simulink model "SF105A_MotCurrRegVltgLimr"  (R2013b)
settings: Solver=FixedStepDiscrete  SolverMode=SingleTasking  StartTime=0.0  StopTime=1  FixedStep=0.00025  RelTol=1e-3
undefined symbols (not defined in the file): ARCHGLBPRM_2OVERSQRT3_ULS_F32, ARCHGLBPRM_2PI_ULS_F32, BRDGVLTGHILIM_VOLT_F32, ELECGLBPRM_PWMPERDNOMX2_SEC_F32, F32TOU16OVR2PI_ULS_F32, MotCurrRegCfgCurrLoopSecOrderTrfFctEna, MotCurrRegCfgMotRVirtDax, MotCurrRegCfgMotRVirtQax, MotCurrRegVltgLimrCurrLoaScarSlewRate, MotCurrRegVltgLimrDaxAntiWdupCoeff, MotCurrRegVltgLimrDualEcuLoaScarSlewRate, MotCurrRegVltgLimrIvtrLoaScarSlewRate, MotCurrRegVltgLimrMotCurrPredEna, MotCurrRegVltgLimrMotCurrPredTi, MotCurrRegVltgLimrMotCurrQaxRefMdfnRplEna, MotCurrRegVltgLimrMotVltgBrdgFilEna, MotCurrRegVltgLimrMotVltgDaxIntglHiLim, MotCurrRegVltgLimrMotVltgDaxIntglLoLim, MotCurrRegVltgLimrMotVltgQaxFfFilEna, MotCurrRegVltgLimrMotVltgQaxIntglHiLim, MotCurrRegVltgLimrMotVltgQaxIntglLoLim, MotCurrRegVltgLimrQaxAntiWdupCoeff, MotCurrRegVltgLimrQaxAntiWdupScagDi, MotRefMdlFbCtrlDi, MotRefMdlIvtrDeadTiBrdgVltgSca, SysSt1, ZERO_VOLT_F32
libraries: NxtrLim x15, Fil x4, simulink x3, NxtrMax x2, NxtrMin x2
(part 5 of 5)

== system SF105A_MotCurrRegVltgLimr/MotCurrRegVltgLimr/MotCurrRegVltgLimrPer1/Kp_Ki_Ctrl_Qax/If Action Subsystem ==
  In1 : Inport
  Action Port : ActionPort  ActionType=then
  CopyRight2 : Subsystem  Description=|  mask(Copyright Information){none=on}
      | Copyright info block.                                               
      |                                                                     
      | Place copyright information at the top of every subsystem in design.
      mask prompts: none "No parameters"
      mask help: Place copyright information at the top of every subsystem in design.
      mask Display:
      | NxtrConf = 'Nexteer Confidential';
      | 
      | sys = bdroot; %handle for the current model ("system")
      | first = get_param(sys,'Created');
      | if(isempty(first))
      |     first = datestr(now,'yyyy');
      | else
      |     first = first(end-3:end);  %year is last four digits
      | end
      | 
      | last = get_param(sys,'LastModifiedDate');
      | if isempty(last)
      |     last = datestr(now,'yyyy');
      | else
      |     last = last(end-3:end);
      | end
      | 
      | if strcmp(first,last)
      |     fprintf('%s -- Copyright %s Nexteer',NxtrConf,first)
      | else
      |     fprintf('%s -- %s%s- %s Nexteer',NxtrConf,char(169),first,last)
      | end
  Out1 : Outport
  wires:
  In1/1 -> Out1/1

== system SF105A_MotCurrRegVltgLimr/MotCurrRegVltgLimr/MotCurrRegVltgLimrPer1/Kp_Ki_Ctrl_Qax/If Action Subsystem1 ==
  In1 : Inport
  Action Port : ActionPort  ActionType=else
  CopyRight2 : Subsystem  Description=|  mask(Copyright Information){none=on}
      | Copyright info block.                                               
      |                                                                     
      | Place copyright information at the top of every subsystem in design.
      mask prompts: none "No parameters"
      mask help: Place copyright information at the top of every subsystem in design.
      mask Display:
      | NxtrConf = 'Nexteer Confidential';
      | 
      | sys = bdroot; %handle for the current model ("system")
      | first = get_param(sys,'Created');
      | if(isempty(first))
      |     first = datestr(now,'yyyy');
      | else
      |     first = first(end-3:end);  %year is last four digits
      | end
      | 
      | last = get_param(sys,'LastModifiedDate');
      | if isempty(last)
      |     last = datestr(now,'yyyy');
      | else
      |     last = last(end-3:end);
      | end
      | 
      | if strcmp(first,last)
      |     fprintf('%s -- Copyright %s Nexteer',NxtrConf,first)
      | else
      |     fprintf('%s -- %s%s- %s Nexteer',NxtrConf,char(169),first,last)
      | end
  Out1 : Outport
  wires:
  In1/1 -> Out1/1

== system SF105A_MotCurrRegVltgLimr/MotCurrRegVltgLimr/MotCurrRegVltgLimrPer1/LOA_ScaFac/CopyRight2 ==

== system SF105A_MotCurrRegVltgLimr/MotCurrRegVltgLimr/MotCurrRegVltgLimrPer1/LOA_ScaFac/If Action Subsystem ==
  In1 : Inport
  Action Port : ActionPort  ActionType=then
  CopyRight2 : Subsystem  Description=|  mask(Copyright Information){none=on}
      | Copyright info block.                                               
      |                                                                     
      | Place copyright information at the top of every subsystem in design.
      mask prompts: none "No parameters"
      mask help: Place copyright information at the top of every subsystem in design.
      mask Display:
      | NxtrConf = 'Nexteer Confidential';
      | 
      | sys = bdroot; %handle for the current model ("system")
      | first = get_param(sys,'Created');
      | if(isempty(first))
      |     first = datestr(now,'yyyy');
      | else
      |     first = first(end-3:end);  %year is last four digits
      | end
      | 
      | last = get_param(sys,'LastModifiedDate');
      | if isempty(last)
      |     last = datestr(now,'yyyy');
      | else
      |     last = last(end-3:end);
      | end
      | 
      | if strcmp(first,last)
      |     fprintf('%s -- Copyright %s Nexteer',NxtrConf,first)
      | else
      |     fprintf('%s -- %s%s- %s Nexteer',NxtrConf,char(169),first,last)
      | end
  Out1 : Outport
  wires:
  In1/1 -> Out1/1

== system SF105A_MotCurrRegVltgLimr/MotCurrRegVltgLimr/MotCurrRegVltgLimrPer1/LOA_ScaFac/If Action Subsystem1 ==
  In1 : Inport
  Action Port : ActionPort  ActionType=else
  CopyRight2 : Subsystem  Description=|  mask(Copyright Information){none=on}
      | Copyright info block.                                               
      |                                                                     
      | Place copyright information at the top of every subsystem in design.
      mask prompts: none "No parameters"
      mask help: Place copyright information at the top of every subsystem in design.
      mask Display:
      | NxtrConf = 'Nexteer Confidential';
      | 
      | sys = bdroot; %handle for the current model ("system")
      | first = get_param(sys,'Created');
      | if(isempty(first))
      |     first = datestr(now,'yyyy');
      | else
      |     first = first(end-3:end);  %year is last four digits
      | end
      | 
      | last = get_param(sys,'LastModifiedDate');
      | if isempty(last)
      |     last = datestr(now,'yyyy');
      | else
      |     last = last(end-3:end);
      | end
      | 
      | if strcmp(first,last)
      |     fprintf('%s -- Copyright %s Nexteer',NxtrConf,first)
      | else
      |     fprintf('%s -- %s%s- %s Nexteer',NxtrConf,char(169),first,last)
      | end
  Out1 : Outport
  wires:
  In1/1 -> Out1/1

== system SF105A_MotCurrRegVltgLimr/MotCurrRegVltgLimr/MotCurrRegVltgLimrPer1/LOA_ScaFac/If Action Subsystem2 ==
  In1 : Inport
  Action Port : ActionPort  ActionType=then
  CopyRight2 : Subsystem  Description=|  mask(Copyright Information){none=on}
      | Copyright info block.                                               
      |                                                                     
      | Place copyright information at the top of every subsystem in design.
      mask prompts: none "No parameters"
      mask help: Place copyright information at the top of every subsystem in design.
      mask Display:
      | NxtrConf = 'Nexteer Confidential';
      | 
      | sys = bdroot; %handle for the current model ("system")
      | first = get_param(sys,'Created');
      | if(isempty(first))
      |     first = datestr(now,'yyyy');
      | else
      |     first = first(end-3:end);  %year is last four digits
      | end
      | 
      | last = get_param(sys,'LastModifiedDate');
      | if isempty(last)
      |     last = datestr(now,'yyyy');
      | else
      |     last = last(end-3:end);
      | end
      | 
      | if strcmp(first,last)
      |     fprintf('%s -- Copyright %s Nexteer',NxtrConf,first)
      | else
      |     fprintf('%s -- %s%s- %s Nexteer',NxtrConf,char(169),first,last)
      | end
  Out1 : Outport
  wires:
  In1/1 -> Out1/1

== system SF105A_MotCurrRegVltgLimr/MotCurrRegVltgLimr/MotCurrRegVltgLimrPer1/LOA_ScaFac/If Action Subsystem3 ==
  In1 : Inport
  Action Port : ActionPort  ActionType=else
  CopyRight2 : Subsystem  Description=|  mask(Copyright Information){none=on}
      | Copyright info block.                                               
      |                                                                     
      | Place copyright information at the top of every subsystem in design.
      mask prompts: none "No parameters"
      mask help: Place copyright information at the top of every subsystem in design.
      mask Display:
      | NxtrConf = 'Nexteer Confidential';
      | 
      | sys = bdroot; %handle for the current model ("system")
      | first = get_param(sys,'Created');
      | if(isempty(first))
      |     first = datestr(now,'yyyy');
      | else
      |     first = first(end-3:end);  %year is last four digits
      | end
      | 
      | last = get_param(sys,'LastModifiedDate');
      | if isempty(last)
      |     last = datestr(now,'yyyy');
      | else
      |     last = last(end-3:end);
      | end
      | 
      | if strcmp(first,last)
      |     fprintf('%s -- Copyright %s Nexteer',NxtrConf,first)
      | else
      |     fprintf('%s -- %s%s- %s Nexteer',NxtrConf,char(169),first,last)
      | end
  Out1 : Outport
  wires:
  In1/1 -> Out1/1

== system SF105A_MotCurrRegVltgLimr/MotCurrRegVltgLimr/MotCurrRegVltgLimrPer1/LOA_ScaFac/If Action Subsystem4 ==
  In1 : Inport
  Action Port : ActionPort  ActionType=then
  CopyRight2 : Subsystem  Description=|  mask(Copyright Information){none=on}
      | Copyright info block.                                               
      |                                                                     
      | Place copyright information at the top of every subsystem in design.
      mask prompts: none "No parameters"
      mask help: Place copyright information at the top of every subsystem in design.
      mask Display:
      | NxtrConf = 'Nexteer Confidential';
      | 
      | sys = bdroot; %handle for the current model ("system")
      | first = get_param(sys,'Created');
      | if(isempty(first))
      |     first = datestr(now,'yyyy');
      | else
      |     first = first(end-3:end);  %year is last four digits
      | end
      | 
      | last = get_param(sys,'LastModifiedDate');
      | if isempty(last)
      |     last = datestr(now,'yyyy');
      | else
      |     last = last(end-3:end);
      | end
      | 
      | if strcmp(first,last)
      |     fprintf('%s -- Copyright %s Nexteer',NxtrConf,first)
      | else
      |     fprintf('%s -- %s%s- %s Nexteer',NxtrConf,char(169),first,last)
      | end
  Out1 : Outport
  wires:
  In1/1 -> Out1/1

== system SF105A_MotCurrRegVltgLimr/MotCurrRegVltgLimr/MotCurrRegVltgLimrPer1/LOA_ScaFac/If Action Subsystem5 ==
  In1 : Inport
  Action Port : ActionPort  ActionType=else
  CopyRight2 : Subsystem  Description=|  mask(Copyright Information){none=on}
      | Copyright info block.                                               
      |                                                                     
      | Place copyright information at the top of every subsystem in design.
      mask prompts: none "No parameters"
      mask help: Place copyright information at the top of every subsystem in design.
      mask Display:
      | NxtrConf = 'Nexteer Confidential';
      | 
      | sys = bdroot; %handle for the current model ("system")
      | first = get_param(sys,'Created');
      | if(isempty(first))
      |     first = datestr(now,'yyyy');
      | else
      |     first = first(end-3:end);  %year is last four digits
      | end
      | 
      | last = get_param(sys,'LastModifiedDate');
      | if isempty(last)
      |     last = datestr(now,'yyyy');
      | else
      |     last = last(end-3:end);
      | end
      | 
      | if strcmp(first,last)
      |     fprintf('%s -- Copyright %s Nexteer',NxtrConf,first)
      | else
      |     fprintf('%s -- %s%s- %s Nexteer',NxtrConf,char(169),first,last)
      | end
  Out1 : Outport
  wires:
  In1/1 -> Out1/1

== system SF105A_MotCurrRegVltgLimr/MotCurrRegVltgLimr/MotCurrRegVltgLimrPer1/MotCurr_ErrCalc_Dax/CopyRight2 ==

== system SF105A_MotCurrRegVltgLimr/MotCurrRegVltgLimr/MotCurrRegVltgLimrPer1/MotCurr_ErrorCalc_Qax/CopyRight2 ==

== system SF105A_MotCurrRegVltgLimr/MotCurrRegVltgLimr/MotCurrRegVltgLimrPer1/MotCurr_ErrorCalc_Qax/If Action Subsystem ==
  In1 : Inport
  Action Port : ActionPort  ActionType=then
  CopyRight2 : Subsystem  Description=|  mask(Copyright Information){none=on}
      | Copyright info block.                                               
      |                                                                     
      | Place copyright information at the top of every subsystem in design.
      mask prompts: none "No parameters"
      mask help: Place copyright information at the top of every subsystem in design.
      mask Display:
      | NxtrConf = 'Nexteer Confidential';
      | 
      | sys = bdroot; %handle for the current model ("system")
      | first = get_param(sys,'Created');
      | if(isempty(first))
      |     first = datestr(now,'yyyy');
      | else
      |     first = first(end-3:end);  %year is last four digits
      | end
      | 
      | last = get_param(sys,'LastModifiedDate');
      | if isempty(last)
      |     last = datestr(now,'yyyy');
      | else
      |     last = last(end-3:end);
      | end
      | 
      | if strcmp(first,last)
      |     fprintf('%s -- Copyright %s Nexteer',NxtrConf,first)
      | else
      |     fprintf('%s -- %s%s- %s Nexteer',NxtrConf,char(169),first,last)
      | end
  Out1 : Outport
  wires:
  In1/1 -> Out1/1

== system SF105A_MotCurrRegVltgLimr/MotCurrRegVltgLimr/MotCurrRegVltgLimrPer1/MotCurr_ErrorCalc_Qax/If Action Subsystem1 ==
  In1 : Inport
  Action Port : ActionPort  ActionType=else
  CopyRight2 : Subsystem  Description=|  mask(Copyright Information){none=on}
      | Copyright info block.                                               
      |                                                                     
      | Place copyright information at the top of every subsystem in design.
      mask prompts: none "No parameters"
      mask help: Place copyright information at the top of every subsystem in design.
      mask Display:
      | NxtrConf = 'Nexteer Confidential';
      | 
      | sys = bdroot; %handle for the current model ("system")
      | first = get_param(sys,'Created');
      | if(isempty(first))
      |     first = datestr(now,'yyyy');
      | else
      |     first = first(end-3:end);  %year is last four digits
      | end
      | 
      | last = get_param(sys,'LastModifiedDate');
      | if isempty(last)
      |     last = datestr(now,'yyyy');
      | else
      |     last = last(end-3:end);
      | end
      | 
      | if strcmp(first,last)
      |     fprintf('%s -- Copyright %s Nexteer',NxtrConf,first)
      | else
      |     fprintf('%s -- %s%s- %s Nexteer',NxtrConf,char(169),first,last)
      | end
  Out1 : Outport
  wires:
  In1/1 -> Out1/1

== system SF105A_MotCurrRegVltgLimr/MotCurrRegVltgLimr/MotCurrRegVltgLimrPer1/MotCurr_Pred/CopyRight2 ==

== system SF105A_MotCurrRegVltgLimr/MotCurrRegVltgLimr/MotCurrRegVltgLimrPer1/MotCurr_Pred/If Action Subsystem2 ==
  In1 : Inport
  Action Port : ActionPort  ActionType=then
  CopyRight2 : Subsystem  Description=|  mask(Copyright Information){none=on}
      | Copyright info block.                                               
      |                                                                     
      | Place copyright information at the top of every subsystem in design.
      mask prompts: none "No parameters"
      mask help: Place copyright information at the top of every subsystem in design.
      mask Display:
      | NxtrConf = 'Nexteer Confidential';
      | 
      | sys = bdroot; %handle for the current model ("system")
      | first = get_param(sys,'Created');
      | if(isempty(first))
      |     first = datestr(now,'yyyy');
      | else
      |     first = first(end-3:end);  %year is last four digits
      | end
      | 
      | last = get_param(sys,'LastModifiedDate');
      | if isempty(last)
      |     last = datestr(now,'yyyy');
      | else
      |     last = last(end-3:end);
      | end
      | 
      | if strcmp(first,last)
      |     fprintf('%s -- Copyright %s Nexteer',NxtrConf,first)
      | else
      |     fprintf('%s -- %s%s- %s Nexteer',NxtrConf,char(169),first,last)
      | end
  Out1 : Outport
  wires:
  In1/1 -> Out1/1

== system SF105A_MotCurrRegVltgLimr/MotCurrRegVltgLimr/MotCurrRegVltgLimrPer1/MotCurr_Pred/If Action Subsystem3 ==
  In1 : Inport
  Action Port : ActionPort  ActionType=else
  CopyRight2 : Subsystem  Description=|  mask(Copyright Information){none=on}
      | Copyright info block.                                               
      |                                                                     
      | Place copyright information at the top of every subsystem in design.
      mask prompts: none "No parameters"
      mask help: Place copyright information at the top of every subsystem in design.
      mask Display:
      | NxtrConf = 'Nexteer Confidential';
      | 
      | sys = bdroot; %handle for the current model ("system")
      | first = get_param(sys,'Created');
      | if(isempty(first))
      |     first = datestr(now,'yyyy');
      | else
      |     first = first(end-3:end);  %year is last four digits
      | end
      | 
      | last = get_param(sys,'LastModifiedDate');
      | if isempty(last)
      |     last = datestr(now,'yyyy');
      | else
      |     last = last(end-3:end);
      | end
      | 
      | if strcmp(first,last)
      |     fprintf('%s -- Copyright %s Nexteer',NxtrConf,first)
      | else
      |     fprintf('%s -- %s%s- %s Nexteer',NxtrConf,char(169),first,last)
      | end
  Out1 : Outport
  wires:
  In1/1 -> Out1/1

== system SF105A_MotCurrRegVltgLimr/MotCurrRegVltgLimr/MotCurrRegVltgLimrPer1/Qax_Vltg_Sum/CopyRight2 ==

== system SF105A_MotCurrRegVltgLimr/MotCurrRegVltgLimr/MotCurrRegVltgLimrPer1/Qax_Vltg_Sum/If Action Subsystem ==
  In1 : Inport
  Action Port : ActionPort  ActionType=then
  CopyRight2 : Subsystem  Description=|  mask(Copyright Information){none=on}
      | Copyright info block.                                               
      |                                                                     
      | Place copyright information at the top of every subsystem in design.
      mask prompts: none "No parameters"
      mask help: Place copyright information at the top of every subsystem in design.
      mask Display:
      | NxtrConf = 'Nexteer Confidential';
      | 
      | sys = bdroot; %handle for the current model ("system")
      | first = get_param(sys,'Created');
      | if(isempty(first))
      |     first = datestr(now,'yyyy');
      | else
      |     first = first(end-3:end);  %year is last four digits
      | end
      | 
      | last = get_param(sys,'LastModifiedDate');
      | if isempty(last)
      |     last = datestr(now,'yyyy');
      | else
      |     last = last(end-3:end);
      | end
      | 
      | if strcmp(first,last)
      |     fprintf('%s -- Copyright %s Nexteer',NxtrConf,first)
      | else
      |     fprintf('%s -- %s%s- %s Nexteer',NxtrConf,char(169),first,last)
      | end
  Out1 : Outport
  wires:
  In1/1 -> Out1/1

== system SF105A_MotCurrRegVltgLimr/MotCurrRegVltgLimr/MotCurrRegVltgLimrPer1/Qax_Vltg_Sum/If Action Subsystem1 ==
  In1 : Inport
  Action Port : ActionPort  ActionType=else
  CopyRight2 : Subsystem  Description=|  mask(Copyright Information){none=on}
      | Copyright info block.                                               
      |                                                                     
      | Place copyright information at the top of every subsystem in design.
      mask prompts: none "No parameters"
      mask help: Place copyright information at the top of every subsystem in design.
      mask Display:
      | NxtrConf = 'Nexteer Confidential';
      | 
      | sys = bdroot; %handle for the current model ("system")
      | first = get_param(sys,'Created');
      | if(isempty(first))
      |     first = datestr(now,'yyyy');
      | else
      |     first = first(end-3:end);  %year is last four digits
      | end
      | 
      | last = get_param(sys,'LastModifiedDate');
      | if isempty(last)
      |     last = datestr(now,'yyyy');
      | else
      |     last = last(end-3:end);
      | end
      | 
      | if strcmp(first,last)
      |     fprintf('%s -- Copyright %s Nexteer',NxtrConf,first)
      | else
      |     fprintf('%s -- %s%s- %s Nexteer',NxtrConf,char(169),first,last)
      | end
  Out1 : Outport
  wires:
  In1/1 -> Out1/1

== system SF105A_MotCurrRegVltgLimr/MotCurrRegVltgLimr/MotCurrRegVltgLimrPer1/VltgSatn_AntiWindup/CopyRight2 ==

== system SF105A_MotCurrRegVltgLimr/MotCurrRegVltgLimr/MotCurrRegVltgLimrPer1/VltgSatn_AntiWindup/If Action Subsystem ==
  In1 : Inport
  Action Port : ActionPort
  CopyRight2 : Subsystem  Description=|  mask(Copyright Information){none=on}
      | Copyright info block.                                               
      |                                                                     
      | Place copyright information at the top of every subsystem in design.
      mask prompts: none "No parameters"
      mask help: Place copyright information at the top of every subsystem in design.
      mask Display:
      | NxtrConf = 'Nexteer Confidential';
      | 
      | sys = bdroot; %handle for the current model ("system")
      | first = get_param(sys,'Created');
      | if(isempty(first))
      |     first = datestr(now,'yyyy');
      | else
      |     first = first(end-3:end);  %year is last four digits
      | end
      | 
      | last = get_param(sys,'LastModifiedDate');
      | if isempty(last)
      |     last = datestr(now,'yyyy');
      | else
      |     last = last(end-3:end);
      | end
      | 
      | if strcmp(first,last)
      |     fprintf('%s -- Copyright %s Nexteer',NxtrConf,first)
      | else
      |     fprintf('%s -- %s%s- %s Nexteer',NxtrConf,char(169),first,last)
      | end
  Out1 : Outport
  wires:
  In1/1 -> Out1/1

== system SF105A_MotCurrRegVltgLimr/MotCurrRegVltgLimr/MotCurrRegVltgLimrPer1/VltgSatn_AntiWindup/If Action Subsystem1 ==
  In1 : Inport
  Action Port : ActionPort
  CopyRight2 : Subsystem  Description=|  mask(Copyright Information){none=on}
      | Copyright info block.                                               
      |                                                                     
      | Place copyright information at the top of every subsystem in design.
      mask prompts: none "No parameters"
      mask help: Place copyright information at the top of every subsystem in design.
      mask Display:
      | NxtrConf = 'Nexteer Confidential';
      | 
      | sys = bdroot; %handle for the current model ("system")
      | first = get_param(sys,'Created');
      | if(isempty(first))
      |     first = datestr(now,'yyyy');
      | else
      |     first = first(end-3:end);  %year is last four digits
      | end
      | 
      | last = get_param(sys,'LastModifiedDate');
      | if isempty(last)
      |     last = datestr(now,'yyyy');
      | else
      |     last = last(end-3:end);
      | end
      | 
      | if strcmp(first,last)
      |     fprintf('%s -- Copyright %s Nexteer',NxtrConf,first)
      | else
      |     fprintf('%s -- %s%s- %s Nexteer',NxtrConf,char(169),first,last)
      | end
  Out1 : Outport
  wires:
  In1/1 -> Out1/1

== system SF105A_MotCurrRegVltgLimr/MotCurrRegVltgLimr/MotCurrRegVltgLimrPer1/Calc_Limit_Cmd_Final/BrdgVltgFiltering/CopyRight1 ==

== system SF105A_MotCurrRegVltgLimr/MotCurrRegVltgLimr/MotCurrRegVltgLimrPer1/Calc_Limit_Cmd_Final/BrdgVltgFiltering/If Action Subsystem ==
  In1 : Inport
  Action Port : ActionPort  ActionType=then
  CopyRight2 : Subsystem  Description=|  mask(Copyright Information){none=on}
      | Copyright info block.                                               
      |                                                                     
      | Place copyright information at the top of every subsystem in design.
      mask prompts: none "No parameters"
      mask help: Place copyright information at the top of every subsystem in design.
      mask Display:
      | NxtrConf = 'Nexteer Confidential';
      | 
      | sys = bdroot; %handle for the current model ("system")
      | first = get_param(sys,'Created');
      | if(isempty(first))
      |     first = datestr(now,'yyyy');
      | else
      |     first = first(end-3:end);  %year is last four digits
      | end
      | 
      | last = get_param(sys,'LastModifiedDate');
      | if isempty(last)
      |     last = datestr(now,'yyyy');
      | else
      |     last = last(end-3:end);
      | end
      | 
      | if strcmp(first,last)
      |     fprintf('%s -- Copyright %s Nexteer',NxtrConf,first)
      | else
      |     fprintf('%s -- %s%s- %s Nexteer',NxtrConf,char(169),first,last)
      | end
  Out1 : Outport
  wires:
  In1/1 -> Out1/1

== system SF105A_MotCurrRegVltgLimr/MotCurrRegVltgLimr/MotCurrRegVltgLimrPer1/Calc_Limit_Cmd_Final/BrdgVltgFiltering/If Action Subsystem1 ==
  In1 : Inport
  Action Port : ActionPort  ActionType=else
  CopyRight2 : Subsystem  Description=|  mask(Copyright Information){none=on}
      | Copyright info block.                                               
      |                                                                     
      | Place copyright information at the top of every subsystem in design.
      mask prompts: none "No parameters"
      mask help: Place copyright information at the top of every subsystem in design.
      mask Display:
      | NxtrConf = 'Nexteer Confidential';
      | 
      | sys = bdroot; %handle for the current model ("system")
      | first = get_param(sys,'Created');
      | if(isempty(first))
      |     first = datestr(now,'yyyy');
      | else
      |     first = first(end-3:end);  %year is last four digits
      | end
      | 
      | last = get_param(sys,'LastModifiedDate');
      | if isempty(last)
      |     last = datestr(now,'yyyy');
      | else
      |     last = last(end-3:end);
      | end
      | 
      | if strcmp(first,last)
      |     fprintf('%s -- Copyright %s Nexteer',NxtrConf,first)
      | else
      |     fprintf('%s -- %s%s- %s Nexteer',NxtrConf,char(169),first,last)
      | end
  Out1 : Outport
  wires:
  In1/1 -> Out1/1

== system SF105A_MotCurrRegVltgLimr/MotCurrRegVltgLimr/MotCurrRegVltgLimrPer1/Calc_Limit_Cmd_Final/PhaAdvCalc/Add 2 Pi ==
  In1 : Inport
  Action Port : ActionPort  ActionType=elseif
  Add : Sum
  Constant : Constant  Value=ARCHGLBPRM_2PI_ULS_F32
  CopyRight2 : Subsystem  Description=|  mask(Copyright Information){none=on}
      | Copyright info block.                                               
      |                                                                     
      | Place copyright information at the top of every subsystem in design.
      mask prompts: none "No parameters"
      mask help: Place copyright information at the top of every subsystem in design.
      mask Display:
      | NxtrConf = 'Nexteer Confidential';
      | 
      | sys = bdroot; %handle for the current model ("system")
      | first = get_param(sys,'Created');
      | if(isempty(first))
      |     first = datestr(now,'yyyy');
      | else
      |     first = first(end-3:end);  %year is last four digits
      | end
      | 
      | last = get_param(sys,'LastModifiedDate');
      | if isempty(last)
      |     last = datestr(now,'yyyy');
      | else
      |     last = last(end-3:end);
      | end
      | 
      | if strcmp(first,last)
      |     fprintf('%s -- Copyright %s Nexteer',NxtrConf,first)
      | else
      |     fprintf('%s -- %s%s- %s Nexteer',NxtrConf,char(169),first,last)
      | end
  Out1 : Outport
  wires:
  In1/1 -> Add/1
  Add/1 -> Out1/1
  Constant/1 -> Add/2

== system SF105A_MotCurrRegVltgLimr/MotCurrRegVltgLimr/MotCurrRegVltgLimrPer1/Calc_Limit_Cmd_Final/PhaAdvCalc/CopyRight2 ==

== system SF105A_MotCurrRegVltgLimr/MotCurrRegVltgLimr/MotCurrRegVltgLimrPer1/Calc_Limit_Cmd_Final/PhaAdvCalc/Do Nothing ==
  In1 : Inport
  Action Port : ActionPort  ActionType=else
  CopyRight2 : Subsystem  Description=|  mask(Copyright Information){none=on}
      | Copyright info block.                                               
      |                                                                     
      | Place copyright information at the top of every subsystem in design.
      mask prompts: none "No parameters"
      mask help: Place copyright information at the top of every subsystem in design.
      mask Display:
      | NxtrConf = 'Nexteer Confidential';
      | 
      | sys = bdroot; %handle for the current model ("system")
      | first = get_param(sys,'Created');
      | if(isempty(first))
      |     first = datestr(now,'yyyy');
      | else
      |     first = first(end-3:end);  %year is last four digits
      | end
      | 
      | last = get_param(sys,'LastModifiedDate');
      | if isempty(last)
      |     last = datestr(now,'yyyy');
      | else
      |     last = last(end-3:end);
      | end
      | 
      | if strcmp(first,last)
      |     fprintf('%s -- Copyright %s Nexteer',NxtrConf,first)
      | else
      |     fprintf('%s -- %s%s- %s Nexteer',NxtrConf,char(169),first,last)
      | end
  Out1 : Outport
  wires:
  In1/1 -> Out1/1

== system SF105A_MotCurrRegVltgLimr/MotCurrRegVltgLimr/MotCurrRegVltgLimrPer1/Calc_Limit_Cmd_Final/PhaAdvCalc/Subtract 2 Pi ==
  In1 : Inport
  Action Port : ActionPort  ActionType=then
  Constant : Constant  Value=ARCHGLBPRM_2PI_ULS_F32
  CopyRight2 : Subsystem  Description=|  mask(Copyright Information){none=on}
      | Copyright info block.                                               
      |                                                                     
      | Place copyright information at the top of every subsystem in design.
      mask prompts: none "No parameters"
      mask help: Place copyright information at the top of every subsystem in design.
      mask Display:
      | NxtrConf = 'Nexteer Confidential';
      | 
      | sys = bdroot; %handle for the current model ("system")
      | first = get_param(sys,'Created');
      | if(isempty(first))
      |     first = datestr(now,'yyyy');
      | else
      |     first = first(end-3:end);  %year is last four digits
      | end
      | 
      | last = get_param(sys,'LastModifiedDate');
      | if isempty(last)
      |     last = datestr(now,'yyyy');
      | else
      |     last = last(end-3:end);
      | end
      | 
      | if strcmp(first,last)
      |     fprintf('%s -- Copyright %s Nexteer',NxtrConf,first)
      | else
      |     fprintf('%s -- %s%s- %s Nexteer',NxtrConf,char(169),first,last)
      | end
  Subtract : Sum  Inputs=+-
  Out1 : Outport
  wires:
  Subtract/1 -> Out1/1
  In1/1 -> Subtract/1
  Constant/1 -> Subtract/2

== system SF105A_MotCurrRegVltgLimr/MotCurrRegVltgLimr/MotCurrRegVltgLimrPer1/Calc_Limit_Cmd_Final/VltgCalcFinal/CopyRight2 ==

== system SF105A_MotCurrRegVltgLimr/MotCurrRegVltgLimr/MotCurrRegVltgLimrPer1/Calc_Limit_Cmd_Final/VltgSatnIvsRatioCalc/CalculateInverse ==
  VltgSatnRatio : Inport
  Action Port : ActionPort  ActionType=then
  CopyRight2 : Subsystem  Description=|  mask(Copyright Information){none=on}
      | Copyright info block.                                               
      |                                                                     
      | Place copyright information at the top of every subsystem in design.
      mask prompts: none "No parameters"
      mask help: Place copyright information at the top of every subsystem in design.
      mask Display:
      | NxtrConf = 'Nexteer Confidential';
      | 
      | sys = bdroot; %handle for the current model ("system")
      | first = get_param(sys,'Created');
      | if(isempty(first))
      |     first = datestr(now,'yyyy');
      | else
      |     first = first(end-3:end);  %year is last four digits
      | end
      | 
      | last = get_param(sys,'LastModifiedDate');
      | if isempty(last)
      |     last = datestr(now,'yyyy');
      | else
      |     last = last(end-3:end);
      | end
      | 
      | if strcmp(first,last)
      |     fprintf('%s -- Copyright %s Nexteer',NxtrConf,first)
      | else
      |     fprintf('%s -- %s%s- %s Nexteer',NxtrConf,char(169),first,last)
      | end
  Math Function : Math  Operator=reciprocal  SaturateOnIntegerOverflow=on
  VltgSatnIvsRatio : Outport
  wires:
  VltgSatnRatio/1 -> Math Function/1
  Math Function/1 -> VltgSatnIvsRatio/1

== system SF105A_MotCurrRegVltgLimr/MotCurrRegVltgLimr/MotCurrRegVltgLimrPer1/Calc_Limit_Cmd_Final/VltgSatnIvsRatioCalc/CopyRight2 ==

== system SF105A_MotCurrRegVltgLimr/MotCurrRegVltgLimr/MotCurrRegVltgLimrPer1/Calc_Limit_Cmd_Final/VltgSatnIvsRatioCalc/If Action Subsystem1 ==
  In1 : Inport
  Action Port : ActionPort  ActionType=else
  CopyRight2 : Subsystem  Description=|  mask(Copyright Information){none=on}
      | Copyright info block.                                               
      |                                                                     
      | Place copyright information at the top of every subsystem in design.
      mask prompts: none "No parameters"
      mask help: Place copyright information at the top of every subsystem in design.
      mask Display:
      | NxtrConf = 'Nexteer Confidential';
      | 
      | sys = bdroot; %handle for the current model ("system")
      | first = get_param(sys,'Created');
      | if(isempty(first))
      |     first = datestr(now,'yyyy');
      | else
      |     first = first(end-3:end);  %year is last four digits
      | end
      | 
      | last = get_param(sys,'LastModifiedDate');
      | if isempty(last)
      |     last = datestr(now,'yyyy');
      | else
      |     last = last(end-3:end);
      | end
      | 
      | if strcmp(first,last)
      |     fprintf('%s -- Copyright %s Nexteer',NxtrConf,first)
      | else
      |     fprintf('%s -- %s%s- %s Nexteer',NxtrConf,char(169),first,last)
      | end
  Out1 : Outport
  wires:
  In1/1 -> Out1/1

== system SF105A_MotCurrRegVltgLimr/MotCurrRegVltgLimr/MotCurrRegVltgLimrPer1/DircFb_VltgCalc/Calculate Direct Feedback/CopyRight2 ==

== system SF105A_MotCurrRegVltgLimr/MotCurrRegVltgLimr/MotCurrRegVltgLimrPer1/DircFb_VltgCalc/Calculate Direct Feedback/Pass Through ==
  In1 : Inport
  In2 : Inport  Port=2
  Action Port : ActionPort  ActionType=then
  CopyRight2 : Subsystem  Description=|  mask(Copyright Information){none=on}
      | Copyright info block.                                               
      |                                                                     
      | Place copyright information at the top of every subsystem in design.
      mask prompts: none "No parameters"
      mask help: Place copyright information at the top of every subsystem in design.
      mask Display:
      | NxtrConf = 'Nexteer Confidential';
      | 
      | sys = bdroot; %handle for the current model ("system")
      | first = get_param(sys,'Created');
      | if(isempty(first))
      |     first = datestr(now,'yyyy');
      | else
      |     first = first(end-3:end);  %year is last four digits
      | end
      | 
      | last = get_param(sys,'LastModifiedDate');
      | if isempty(last)
      |     last = datestr(now,'yyyy');
      | else
      |     last = last(end-3:end);
      | end
      | 
      | if strcmp(first,last)
      |     fprintf('%s -- Copyright %s Nexteer',NxtrConf,first)
      | else
      |     fprintf('%s -- %s%s- %s Nexteer',NxtrConf,char(169),first,last)
      | end
  Out1 : Outport
  Out2 : Outport  Port=2
  wires:
  In1/1 -> Out1/1
  In2/1 -> Out2/1

== system SF105A_MotCurrRegVltgLimr/MotCurrRegVltgLimr/MotCurrRegVltgLimrPer1/DircFb_VltgCalc/Calculate Direct Feedback/Pass Through 1 ==
  In1 : Inport
  In2 : Inport  Port=2
  Action Port : ActionPort  ActionType=else
  CopyRight2 : Subsystem  Description=|  mask(Copyright Information){none=on}
      | Copyright info block.                                               
      |                                                                     
      | Place copyright information at the top of every subsystem in design.
      mask prompts: none "No parameters"
      mask help: Place copyright information at the top of every subsystem in design.
      mask Display:
      | NxtrConf = 'Nexteer Confidential';
      | 
      | sys = bdroot; %handle for the current model ("system")
      | first = get_param(sys,'Created');
      | if(isempty(first))
      |     first = datestr(now,'yyyy');
      | else
      |     first = first(end-3:end);  %year is last four digits
      | end
      | 
      | last = get_param(sys,'LastModifiedDate');
      | if isempty(last)
      |     last = datestr(now,'yyyy');
      | else
      |     last = last(end-3:end);
      | end
      | 
      | if strcmp(first,last)
      |     fprintf('%s -- Copyright %s Nexteer',NxtrConf,first)
      | else
      |     fprintf('%s -- %s%s- %s Nexteer',NxtrConf,char(169),first,last)
      | end
  Out1 : Outport
  Out2 : Outport  Port=2
  wires:
  In1/1 -> Out1/1
  In2/1 -> Out2/1

== system SF105A_MotCurrRegVltgLimr/MotCurrRegVltgLimr/MotCurrRegVltgLimrPer1/DircFb_VltgCalc/Zero Direct Feedback/CopyRight2 ==

== system SF105A_MotCurrRegVltgLimr/MotCurrRegVltgLimr/MotCurrRegVltgLimrPer1/Kp_Ki_Ctrl_Dax/If Action Subsystem/CopyRight2 ==

== system SF105A_MotCurrRegVltgLimr/MotCurrRegVltgLimr/MotCurrRegVltgLimrPer1/Kp_Ki_Ctrl_Dax/If Action Subsystem1/CopyRight2 ==

== system SF105A_MotCurrRegVltgLimr/MotCurrRegVltgLimr/MotCurrRegVltgLimrPer1/Kp_Ki_Ctrl_Qax/If Action Subsystem/CopyRight2 ==

== system SF105A_MotCurrRegVltgLimr/MotCurrRegVltgLimr/MotCurrRegVltgLimrPer1/Kp_Ki_Ctrl_Qax/If Action Subsystem1/CopyRight2 ==

== system SF105A_MotCurrRegVltgLimr/MotCurrRegVltgLimr/MotCurrRegVltgLimrPer1/LOA_ScaFac/If Action Subsystem/CopyRight2 ==

== system SF105A_MotCurrRegVltgLimr/MotCurrRegVltgLimr/MotCurrRegVltgLimrPer1/LOA_ScaFac/If Action Subsystem1/CopyRight2 ==

== system SF105A_MotCurrRegVltgLimr/MotCurrRegVltgLimr/MotCurrRegVltgLimrPer1/LOA_ScaFac/If Action Subsystem2/CopyRight2 ==

== system SF105A_MotCurrRegVltgLimr/MotCurrRegVltgLimr/MotCurrRegVltgLimrPer1/LOA_ScaFac/If Action Subsystem3/CopyRight2 ==

== system SF105A_MotCurrRegVltgLimr/MotCurrRegVltgLimr/MotCurrRegVltgLimrPer1/LOA_ScaFac/If Action Subsystem4/CopyRight2 ==

== system SF105A_MotCurrRegVltgLimr/MotCurrRegVltgLimr/MotCurrRegVltgLimrPer1/LOA_ScaFac/If Action Subsystem5/CopyRight2 ==

== system SF105A_MotCurrRegVltgLimr/MotCurrRegVltgLimr/MotCurrRegVltgLimrPer1/MotCurr_ErrorCalc_Qax/If Action Subsystem/CopyRight2 ==

== system SF105A_MotCurrRegVltgLimr/MotCurrRegVltgLimr/MotCurrRegVltgLimrPer1/MotCurr_ErrorCalc_Qax/If Action Subsystem1/CopyRight2 ==

== system SF105A_MotCurrRegVltgLimr/MotCurrRegVltgLimr/MotCurrRegVltgLimrPer1/MotCurr_Pred/If Action Subsystem2/CopyRight2 ==

== system SF105A_MotCurrRegVltgLimr/MotCurrRegVltgLimr/MotCurrRegVltgLimrPer1/MotCurr_Pred/If Action Subsystem3/CopyRight2 ==

== system SF105A_MotCurrRegVltgLimr/MotCurrRegVltgLimr/MotCurrRegVltgLimrPer1/Qax_Vltg_Sum/If Action Subsystem/CopyRight2 ==

== system SF105A_MotCurrRegVltgLimr/MotCurrRegVltgLimr/MotCurrRegVltgLimrPer1/Qax_Vltg_Sum/If Action Subsystem1/CopyRight2 ==

== system SF105A_MotCurrRegVltgLimr/MotCurrRegVltgLimr/MotCurrRegVltgLimrPer1/VltgSatn_AntiWindup/If Action Subsystem/CopyRight2 ==

== system SF105A_MotCurrRegVltgLimr/MotCurrRegVltgLimr/MotCurrRegVltgLimrPer1/VltgSatn_AntiWindup/If Action Subsystem1/CopyRight2 ==

== system SF105A_MotCurrRegVltgLimr/MotCurrRegVltgLimr/MotCurrRegVltgLimrPer1/Calc_Limit_Cmd_Final/BrdgVltgFiltering/If Action Subsystem/CopyRight2 ==

== system SF105A_MotCurrRegVltgLimr/MotCurrRegVltgLimr/MotCurrRegVltgLimrPer1/Calc_Limit_Cmd_Final/BrdgVltgFiltering/If Action Subsystem1/CopyRight2 ==

== system SF105A_MotCurrRegVltgLimr/MotCurrRegVltgLimr/MotCurrRegVltgLimrPer1/Calc_Limit_Cmd_Final/PhaAdvCalc/Add 2 Pi/CopyRight2 ==

== system SF105A_MotCurrRegVltgLimr/MotCurrRegVltgLimr/MotCurrRegVltgLimrPer1/Calc_Limit_Cmd_Final/PhaAdvCalc/Do Nothing/CopyRight2 ==

== system SF105A_MotCurrRegVltgLimr/MotCurrRegVltgLimr/MotCurrRegVltgLimrPer1/Calc_Limit_Cmd_Final/PhaAdvCalc/Subtract 2 Pi/CopyRight2 ==

== system SF105A_MotCurrRegVltgLimr/MotCurrRegVltgLimr/MotCurrRegVltgLimrPer1/Calc_Limit_Cmd_Final/VltgSatnIvsRatioCalc/CalculateInverse/CopyRight2 ==

== system SF105A_MotCurrRegVltgLimr/MotCurrRegVltgLimr/MotCurrRegVltgLimrPer1/Calc_Limit_Cmd_Final/VltgSatnIvsRatioCalc/If Action Subsystem1/CopyRight2 ==

== system SF105A_MotCurrRegVltgLimr/MotCurrRegVltgLimr/MotCurrRegVltgLimrPer1/DircFb_VltgCalc/Calculate Direct Feedback/Pass Through/CopyRight2 ==

== system SF105A_MotCurrRegVltgLimr/MotCurrRegVltgLimr/MotCurrRegVltgLimrPer1/DircFb_VltgCalc/Calculate Direct Feedback/Pass Through 1/CopyRight2 ==
